simulink model "RPC2_state_feedback"  (R2020b)
settings: Solver=ode45  StartTime=0.0  StopTime=100  RelTol=1e-8  AbsTol=1e-10  EnableMultiTasking=on
values from neighbouring files (symbols this model uses):
  A = [0 1 ... (first row only)    [TestDIST_EFFECT_DCmotor_zp(1).m]    (also in TestDIST_EFFECT_DCmotor_zp.m; lqr_DOB_2_5.mat = [0  1; 0  0]; lqr_DOB_5.mat = [0  1; 0  0]; lqr_DOB_8.mat = [0  1; 0  0])
  B = [0; Kt/Rm/Jt]    [TestDIST_EFFECT_DCmotor_zp(1).m]    (also in TestDIST_EFFECT_DCmotor_zp.m; lqr_DOB_2_5.mat = [0 239.250934036]; lqr_DOB_5.mat = [0 239.250934036]; lqr_DOB_8.mat = [0 239.250934036])
  d = [1 -1.75526480336 0.782027160212]    [lqr_DOB_2_5.mat]    (also in lqr_DOB_5.mat; lqr_DOB_8.mat; lqr_noDOB_10.mat = [1 -1.7546251878 0.781376862182]; lqr_noDOB_2_5.mat = [1 -1.7546251878 0.781376862182])
  K = KK    [TestDIST_EFFECT_DCmotor_zp.m]    (also in lqr_DOB_2_5.mat = [27.9647466006 0.483496818901]; lqr_DOB_5.mat = [27.9647466006 0.483496818901]; lqr_DOB_8.mat = [27.9647466006 0.483496818901]; lqr_noDOB_10.mat = [28.2374499722 0.447372514694])
  n = n(2:3)    [TestDIST_EFFECT_DCmotor_zp(1).m]    (also in TestDIST_EFFECT_DCmotor_zp.m; lqr_DOB_2_5.mat = [0.0133811834885 0.0133811834885]; lqr_DOB_5.mat = [0.0133811834885 0.0133811834885]; lqr_DOB_8.mat = [0.0133811834885 0.0133811834885])
settings Model: Creator=oboe  LastModifiedBy=Lab-Mec
settings SolverCC: AutoScaleAbsTol=off
settings DataIOCC: LimitDataPoints=on  SaveFormat=Array  ReturnWorkspaceOutputs=off
settings OptimizationCC: LifeSpan=inf
settings DebuggingCC: SolverPrmCheckMsg=warning  SFUnexpectedBacktrackingDiag=warning  SFNoUnconditionalDefaultTransitionDiag=warning  SFExecutionAtInitializationDiag=none  ArithmeticOperatorsInVariantConditions=warning
settings HardwareCC: ProdBitPerPointer=32  ProdBitPerSizeT=32  ProdBitPerPtrDiffT=32  ProdLargestAtomicFloat=None  ProdIntDivRoundTo=Undefined  ProdEndianess=Unspecified  ProdWordSize=32  ProdHWDeviceType=32-bit Generic
settings ModelReferenceCC: PropagateSignalLabelsOutOfModel=off
settings SFSimCC: SimUseLocalCustomCode=off  CustomCodeUndefinedFunction=UseInterfaceOnly
settings RTWCC: RTWUseLocalCustomCode=off
settings CodeAppCC: StateflowObjectComments=on
settings GRTTargetCC: TargetLangStandard=C89/C90 (ANSI)
settings ConfigComp: CovMetricSettings=dw  CovSaveCumulativeToWorkspaceVar=on  CovSaveSingleToWorkspaceVar=on  CovExternalEMLEnable=off  CovSFcnEnable=off

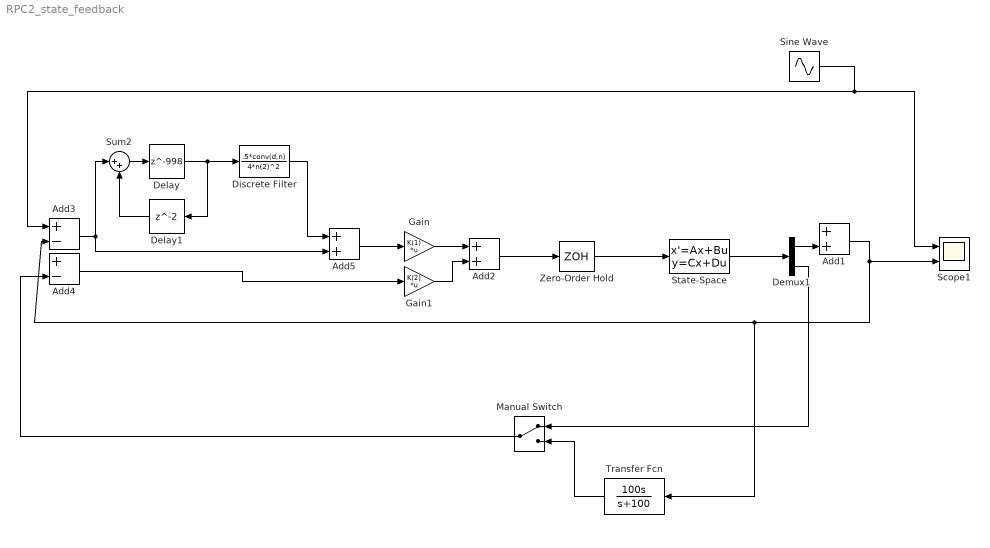
== system RPC2_state_feedback ==
  Add1 : Sum
  Add2 : Sum
  Add3 : Sum  Inputs=+-
  Add4 : Sum  Inputs=+-
  Add5 : Sum
  Delay : Delay  DelayLength=998  UseCircularBuffer=on  SampleTime=.002
  Delay1 : Delay  UseCircularBuffer=on  SampleTime=.002
  Demux1 : Demux  Outputs=2
  Discrete Filter : DiscreteFilter  Numerator=.5*conv(d,n)  Denominator=4*n(2)^2  SampleTime=.002
  Gain : Gain  Gain=K(1)  Multiplication=Matrix(K*u)
  Gain1 : Gain  Gain=K(2)  Multiplication=Matrix(K*u)
  Manual Switch : ManualSwitch
  Scope1 : Scope  NumInputPorts=2
  Sine Wave : Sin  SineType=Sample based  Amplitude=0.1  Samples=500  SampleTime=.002
  State-Space : StateSpace  A=A(1:2,1:2)  B=B(1:2)  C=eye(2)  D=[0;0]  InitialCondition=0
  Sum2 : Sum  Inputs=|++
  Transfer Fcn : TransferFcn  Numerator=[100 0]  Denominator=[1 100]
  Zero-Order Hold : ZeroOrderHold  SampleTime=0.002
  wires:
  Zero-Order Hold/1 -> State-Space/1
  Add1/1 -> Add3/2, Transfer Fcn/1, Scope1/2
  Gain/1 -> Add2/1
  Add2/1 -> Zero-Order Hold/1
  Gain1/1 -> Add2/2
  State-Space/1 -> Demux1/1
  Demux1/1 -> Add1/2
  Sine Wave/1 -> Scope1/1, Add3/1
  Add4/1 -> Gain1/1
  Add5/1 -> Gain/1
  Sum2/1 -> Delay/1
  Delay1/1 -> Sum2/2
  Delay/1 -> Delay1/1, Discrete Filter/1
  Add3/1 -> Add5/2, Sum2/1
  Discrete Filter/1 -> Add5/1
  Transfer Fcn/1 -> Manual Switch/2
  Demux1/2 -> Manual Switch/1
  Manual Switch/1 -> Add4/2
